simulink model "TOAD_simulation"  (R2018b)
settings: Solver=FixedStepAuto  StartTime=0.0  StopTime=tempoS.data(3)  FixedStep=0.05  RelTol=1e-3
values from neighbouring files (symbols this model uses):
  centri_circonferenzeS = timeseries([circonferenza1.centro; circonferenza2.centro])    [main.m]
  phiS = timeseries([phi.iniziale, phi.finale])    [main.m]
  puntoS = timeseries([punto.iniziale; punto.finale])    [main.m]
  raggi_circonferenzeS = timeseries([circonferenza1.raggio; circonferenza2.raggio])    [main.m]
  tempoS = timeseries([tempo.iniziale; tempo.finale1; tempo.finale2])    [main.m]
settings Model: Creator=camillo  LastModifiedBy=camillo

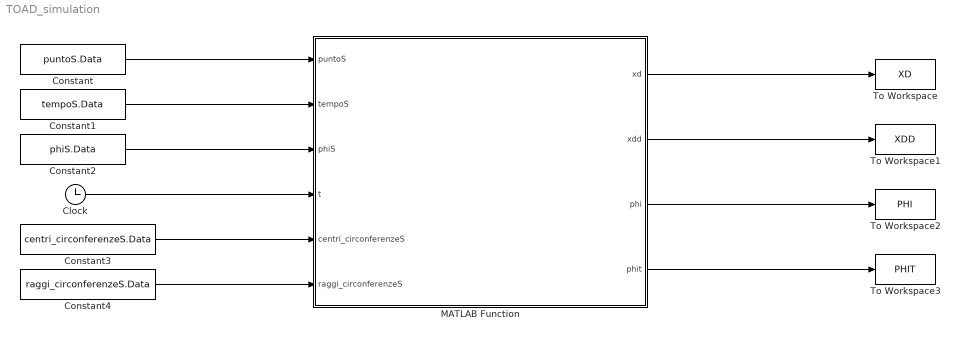
== system TOAD_simulation ==
  Clock : Clock
  Constant : Constant  Value=puntoS.Data
  Constant1 : Constant  Value=tempoS.Data
  Constant2 : Constant  Value=phiS.Data
  Constant3 : Constant  Value=centri_circonferenzeS.Data
  Constant4 : Constant  Value=raggi_circonferenzeS.Data
  MATLAB Function : MATLAB Function  TreatAsAtomicUnit=on
  To Workspace : ToWorkspace  VariableName=XD  SampleTime=-1
  To Workspace1 : ToWorkspace  VariableName=XDD  SampleTime=-1
  To Workspace2 : ToWorkspace  VariableName=PHI  SampleTime=-1
  To Workspace3 : ToWorkspace  VariableName=PHIT  SampleTime=-1
  wires:
  Clock/1 -> MATLAB Function/4(t)
  MATLAB Function/1(xd) -> To Workspace/1
  MATLAB Function/2(xdd) -> To Workspace1/1
  MATLAB Function/3(phi) -> To Workspace2/1
  MATLAB Function/4(phit) -> To Workspace3/1
  Constant/1 -> MATLAB Function/1(puntoS)
  Constant1/1 -> MATLAB Function/2(tempoS)
  Constant2/1 -> MATLAB Function/3(phiS)
  Constant3/1 -> MATLAB Function/5(centri_circonferenzeS)
  Constant4/1 -> MATLAB Function/6(raggi_circonferenzeS)

== matlab function TOAD_simulation/MATLAB Function ==
  data: puntoS input; xd output; tempoS input; phiS input; t input; centri_circonferenzeS input; raggi_circonferenzeS input; xdd output; phi output; phit output
function [xd,xdd,phi,phit] = fcn(puntoS, tempoS, phiS, t, centri_circonferenzeS, raggi_circonferenzeS)

    punto = struct;
    punto.iniziale = puntoS(1,:);
    punto.finale = puntoS(2,:);
    
    tempo = struct;
    tempo.iniziale = tempoS(1);
    tempo.finale1 = tempoS(2);
    tempo.finale2 = tempoS(3);
    
    phi_in = struct;
    phi_in.iniziale = phiS(1);
    phi_in.finale = phiS(2);
    
    circonferenza1 = struct;
    circonferenza1.centro = centri_circonferenzeS(1,:);
    circonferenza1.raggio = raggi_circonferenzeS(1,:);
    
    circonferenza2.centro = centri_circonferenzeS(2,:);
    circonferenza2.raggio = raggi_circonferenzeS(2,:);


    [xd, xdd, phi, phit] = planner_TOAD(punto, tempo, phi_in, t, circonferenza1, circonferenza2);
    
end
